simulink model "task5_6_new"  (R2020b)
settings: Solver=FixedStepAuto  StartTime=0.0  StopTime=90.0  FixedStep=0.01  RelTol=1e-3
settings Model: Creator=hauss  LastModifiedBy=carle

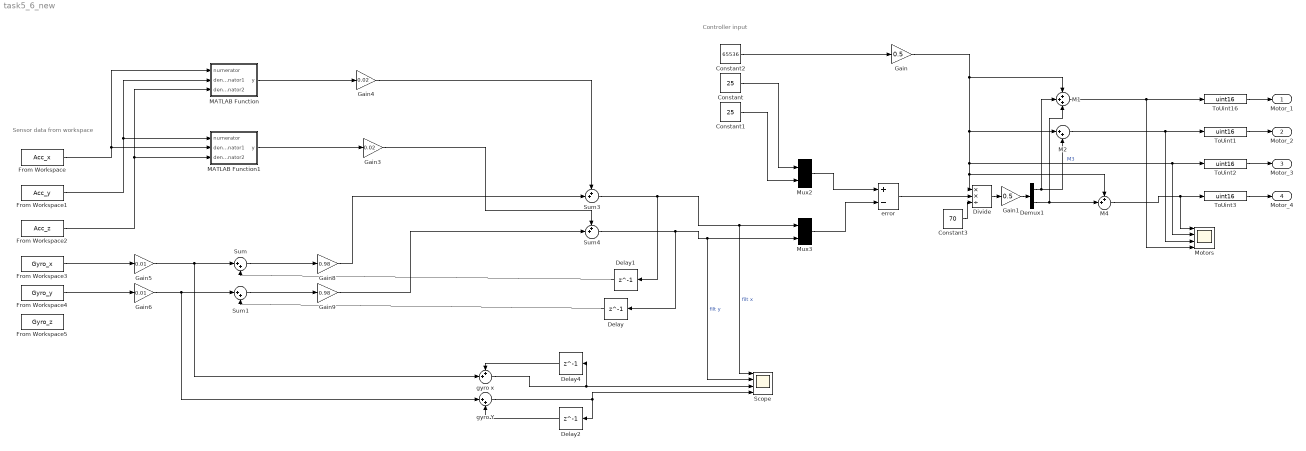
== system task5_6_new ==
  note: Sensor data from
      | workspace
  note: Controller input
  Constant : Constant  Value=25  VectorParams1D=off  SampleTime=90
  Constant1 : Constant  Value=25  VectorParams1D=off  SampleTime=90
  Constant2 : Constant  Value=65536  SampleTime=90
  Constant3 : Constant  Value=70
  Delay{,1..2,4} (4 alike) : Delay  DelayLength=1  InitialCondition=0
  Demux1 : Demux  Outputs=2
  Divide : Product  Inputs=**/
  From Workspace : FromWorkspace  VariableName=Acc_x
  From Workspace1 : FromWorkspace  VariableName=Acc_y
  From Workspace2 : FromWorkspace  VariableName=Acc_z
  From Workspace3 : FromWorkspace  VariableName=Gyro_x
  From Workspace4 : FromWorkspace  VariableName=Gyro_y
  From Workspace5 : FromWorkspace  VariableName=Gyro_z
  Gain : Gain  Gain=0.5
  Gain1 : Gain  Gain=0.5
  Gain3 : Gain  Gain=0.02
  Gain4 : Gain  Gain=0.02
  Gain5 : Gain  Gain=0.01
  Gain6 : Gain  Gain=0.01
  Gain8 : Gain  Gain=0.98
  Gain9 : Gain  Gain=0.98
  M1 : Sum  Inputs=+++
  M2 : Sum  Inputs=|++
  M4 : Sum  Inputs=++|
  MATLAB Function : MATLAB Function  TreatAsAtomicUnit=on
  MATLAB Function1 : MATLAB Function  TreatAsAtomicUnit=on
  Motors : Scope  NumInputPorts=4
  Mux2 : Mux  Inputs=2
  Mux3 : Mux  Inputs=2
  Scope : Scope  NumInputPorts=4
  Sum : Sum  Inputs=|++
  Sum1 : Sum  Inputs=|++
  Sum3 : Sum  Inputs=++|
  Sum4 : Sum  Inputs=++|
  ToUint{1..3,16} (4 alike) : DataTypeConversion  OutDataTypeStr=uint16  SaturateOnIntegerOverflow=on
  error : Sum  Inputs=+-
  gyro Y : Sum  Inputs=|++
  gyro x : Sum  Inputs=++|
  Motor_1 : Outport  OutDataTypeStr=uint16  VectorParamsAs1DForOutWhenUnconnected=off  LockScale=on
  Motor_2 : Outport  Port=2  OutDataTypeStr=uint16  VectorParamsAs1DForOutWhenUnconnected=off  LockScale=on
  Motor_3 : Outport  Port=3  OutDataTypeStr=uint16  VectorParamsAs1DForOutWhenUnconnected=off  LockScale=on
  Motor_4 : Outport  Port=4  OutDataTypeStr=uint16  VectorParamsAs1DForOutWhenUnconnected=off  LockScale=on
  wires:
  Mux2/1 -> error/1
  Constant1/1 -> Mux2/2
  ToUint16/1 -> Motor_1/1
  ToUint1/1 -> Motor_2/1
  ToUint2/1 -> Motor_3/1
  ToUint3/1 -> Motor_4/1
  Constant2/1 -> Gain/1
  error/1 -> Divide/2
  Constant/1 -> Mux2/1
  Mux3/1 -> error/2
  Constant3/1 -> Divide/3
  M2/1 -> Motors/3, ToUint1/1
  Gain/1 -> M2/1, Motors/2, ToUint2/1, M4/1, Divide/1, M1/1  "M3"
  M1/1 -> Motors/4, ToUint16/1
  Demux1/1 -> M2/2, M1/2
  Demux1/2 -> M1/3, M4/2
  M4/1 -> Motors/1, ToUint3/1
  Gain1/1 -> Demux1/1
  Divide/1 -> Gain1/1
  From Workspace/1 -> MATLAB Function/1(numerator), MATLAB Function1/2(denominator1)
  From Workspace1/1 -> MATLAB Function1/1(numerator), MATLAB Function/2(denominator1)
  From Workspace2/1 -> MATLAB Function1/3(denominator2), MATLAB Function/3(denominator2)
  MATLAB Function1/1(y) -> Gain3/1
  MATLAB Function/1(y) -> Gain4/1
  From Workspace3/1 -> Gain5/1
  From Workspace4/1 -> Gain6/1
  Gain6/1 -> gyro Y/1, Sum1/1
  Sum/1 -> Gain8/1
  Sum1/1 -> Gain9/1
  Gain4/1 -> Sum3/1
  Gain8/1 -> Sum3/2
  Gain9/1 -> Sum4/2
  Gain3/1 -> Sum4/1
  Sum4/1 -> Delay/1, Scope/2, Mux3/2  "filt y"
  Delay/1 -> Sum1/2
  Delay1/1 -> Sum/2
  Sum3/1 -> Delay1/1, Scope/1, Mux3/1  "filt x"
  Delay2/1 -> gyro Y/2
  gyro Y/1 -> Scope/4, Delay2/1
  gyro x/1 -> Scope/3, Delay4/1
  Gain5/1 -> gyro x/2, Sum/1
  Delay4/1 -> gyro x/1

== matlab function task5_6_new/MATLAB Function ==
  data: numerator input; y output; denominator1 input; denominator2 input
function y = fcn(numerator,denominator1,denominator2)
    
y = atan2(numerator, sqrt(denominator1^2 + denominator2^2));

== matlab function task5_6_new/MATLAB Function1 ==
  data: numerator input; y output; denominator1 input; denominator2 input
function y = fcn(numerator,denominator1,denominator2)
    
y = atan2(numerator, sqrt(denominator1^2 + denominator2^2));
